simulink model "example"  (R2020a)
settings: Solver=VariableStepAuto  StartTime=0.0  StopTime=stoptime  RelTol=1e-3
values from neighbouring files (symbols this model uses):
  Input_th = [pi/4 0]    [data.m]
libraries: dspfdesign x5
settings Model: Creator=SURAJ  LastModifiedBy=shita
settings DataIOCC: ReturnWorkspaceOutputs=off
settings DebuggingCC: ArithmeticOperatorsInVariantConditions=warning
settings SFSimCC: SimUseLocalCustomCode=off  CustomCodeUndefinedFunction=UseInterfaceOnly
settings RTWCC: RTWUseLocalCustomCode=off

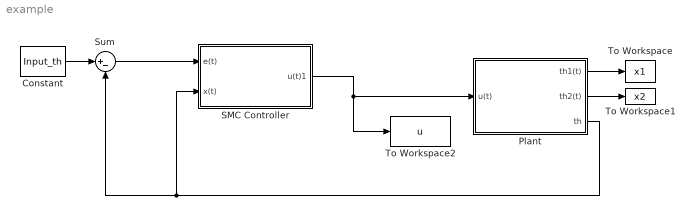
== system example ==
  Constant : Constant  Value=Input_th
  Plant : Subsystem
  SMC Controller : Subsystem
  Sum : Sum  Inputs=|+-
  To Workspace : ToWorkspace  VariableName=x1  SaveFormat=Timeseries  SampleTime=-1
  To Workspace1 : ToWorkspace  VariableName=x2  SaveFormat=Timeseries  SampleTime=-1
  To Workspace2 : ToWorkspace  VariableName=u  SaveFormat=Timeseries  SampleTime=-1
  wires:
  Plant/3(th) -> Sum/2, SMC Controller/2(x(t))
  Plant/1(th1(t)) -> To Workspace/1
  Plant/2(th2(t)) -> To Workspace1/1
  SMC Controller/1(u(t)1) -> To Workspace2/1, Plant/1(u(t))
  Constant/1 -> Sum/1
  Sum/1 -> SMC Controller/1(e(t))

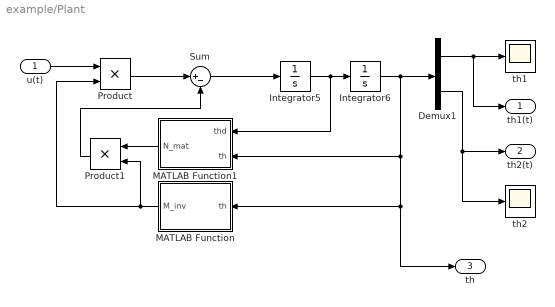
== system example/Plant ==
  u(t) : Inport
  Demux1 : Demux  Outputs=2
  Integrator5 : Integrator
  Integrator6 : Integrator
  MATLAB Function : MATLAB Function  TreatAsAtomicUnit=on
  MATLAB Function1 : MATLAB Function  TreatAsAtomicUnit=on
  Product : Product
  Product1 : Product
  Sum : Sum  Inputs=|+-
  th1 : Scope
  th2 : Scope
  th1(t) : Outport  VectorParamsAs1DForOutWhenUnconnected=off
  th2(t) : Outport  Port=2  VectorParamsAs1DForOutWhenUnconnected=off
  th : Outport  Port=3  VectorParamsAs1DForOutWhenUnconnected=off
  wires:
  u(t)/1 -> Product/1
  Sum/1 -> Integrator5/1
  Demux1/1 -> th1(t)/1, th1/1
  Product1/1 -> Sum/2
  MATLAB Function1/1(N_mat) -> Product1/1
  MATLAB Function/1(M_inv) -> Product1/2, Product/2
  Integrator6/1 -> th/1, MATLAB Function/1(th), MATLAB Function1/2(th), Demux1/1
  Product/1 -> Sum/1
  Demux1/2 -> th2(t)/1, th2/1
  Integrator5/1 -> Integrator6/1, MATLAB Function1/1(thd)

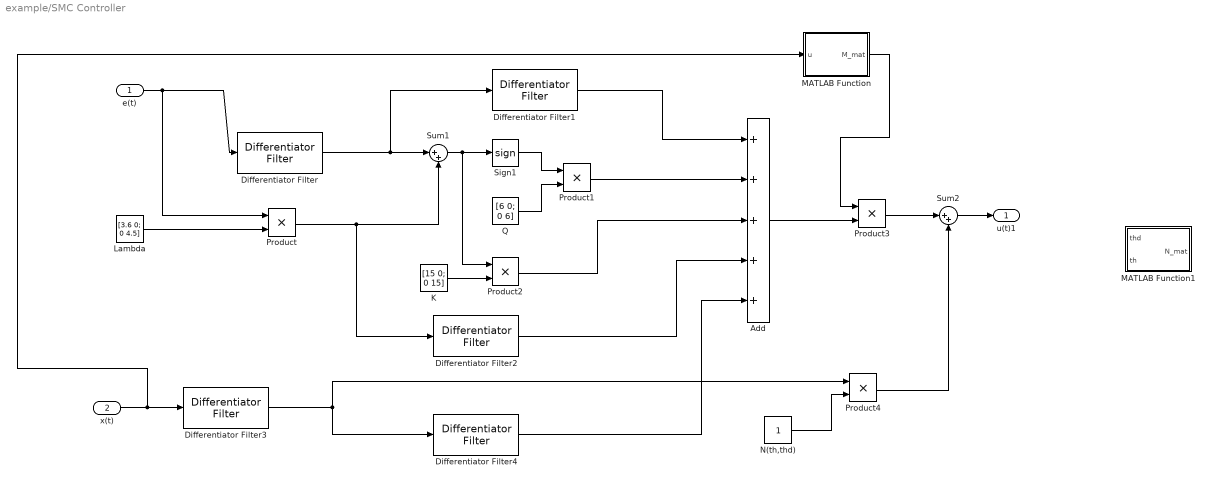
== system example/SMC Controller ==
  e(t) : Inport
  x(t) : Inport  Port=2
  Add : Sum  Inputs=+++++
  Differentiator Filter{,1..4} (5 alike) : dspfdesign/Differentiator Filter  DesignForMinimumOrder=on  FilterOrder=31  PassbandRipple=0.1  ScaleCoefficients=off  SimulateUsing=Interpreted execution  roundingMode=Floor  coeffsDataTypeStr=fixdt(1,16)
      settings: SourceProductBaseCode=DS
  K : Constant  Value=[15 0; 0 15]  VectorParams1D=off
  Lambda : Constant  Value=[3.6 0; 0 4.5]  VectorParams1D=off
  MATLAB Function : MATLAB Function  TreatAsAtomicUnit=on
  MATLAB Function1 : MATLAB Function  TreatAsAtomicUnit=on
  N(th,thd) : Constant
  Product{,1..4} (5 alike) : Product
  Q : Constant  Value=[6 0; 0 6]  VectorParams1D=off
  Sign1 : Signum  ZeroCross=off
  Sum1 : Sum  Inputs=|++
  Sum2 : Sum  Inputs=|++
  u(t)1 : Outport  VectorParamsAs1DForOutWhenUnconnected=off
  wires:
  Differentiator Filter/1 -> Differentiator Filter1/1, Sum1/1
  e(t)/1 -> Differentiator Filter/1, Product/1
  Lambda/1 -> Product/2
  Differentiator Filter1/1 -> Add/1
  Sum1/1 -> Product2/1, Sign1/1
  Sign1/1 -> Product1/1
  Product1/1 -> Add/2
  Q/1 -> Product1/2
  Product/1 -> Differentiator Filter2/1, Sum1/2
  K/1 -> Product2/2
  Product2/1 -> Add/3
  Differentiator Filter2/1 -> Add/4
  Add/1 -> Product3/2
  MATLAB Function/1(M_mat) -> Product3/1
  x(t)/1 -> Differentiator Filter3/1, MATLAB Function/1(u)
  Differentiator Filter3/1 -> Product4/1, Differentiator Filter4/1
  N(th,thd)/1 -> Product4/2
  Product4/1 -> Sum2/2
  Differentiator Filter4/1 -> Add/5
  Product3/1 -> Sum2/1
  Sum2/1 -> u(t)1/1

== matlab function example/SMC Controller/MATLAB Function ==
  data: u input; M_mat output
function M_mat = Mass_mat(u)
m1 = 20;
m2 = 10;
L1 = 0.5;
L2 = 0.5;
a1 = 0.5;
a2 = 0.5;
I1 = 0.8;
I2 = 0.2;
th2 = u(2);
M11 = I1 + m1*L1*L1 + I2 + m2*(a1*a1 + L2*L2 + 2*a1 * L2 * cos(th2));
M12 = I2 + m2 * (L2 * L2 + a1 * L2 * cos(th2));
M21 = M12;
M22 = I2 + m2*L2*L2;
M_mat = [M11 M12; M21 M22];

== matlab function example/Plant/MATLAB Function ==
  data: th input; M_inv output
function M_inv = Mass_mat(th)
th2 = th(2);
m1 = 20;
m2 = 10;
L1 = 0.5;
L2 = 0.5;
a1 = 0.5;
a2 = 0.5;
I1 = 0.8;
I2 = 0.2;
M11 = I1 + m1*L1*L1 + I2 + m2*(a1*a1 + L2*L2 + 2*a1 * L2 * cos(th2));
M12 = I2 + m2 * (L2 * L2 + a1 * L2 * cos(th2));
M21 = M12;
M22 = I2 + m2*L2*L2;
M_mat = [M11 M12; M21 M22];
M_inv = inv(M_mat);

== matlab function example/Plant/MATLAB Function1 ==
  data: thd input; th input; N_mat output
function N_mat= N_func(thd, th)
th1 = th(1);
th2 = th(2);
th1d = thd(1);
th2d = thd(2);
m1 = 20;
m2 = 10;
L1 = 0.5;
L2 = 0.5;
a1 = 0.5;
a2 = 0.5;
N11 = -m2 * a2 * L2 * th1d * sin(th2);
N12 = -m2* a1 * L2*(th1d + th2d)*sin(th2);
N21 = m2*a1*th1d*sin(th2);
N_mat = [(N11*th1d)+(N12*th2d) N21*(th1d)];

== matlab function example/SMC Controller/MATLAB Function1 ==
  data: thd input; N_mat output; th input
function N_mat= N_func(thd, th)
th1 = th(1);
th2 = th(2);
th1d = thd(1);
th2d = thd(2);
m1 = 20;
m2 = 10;
L1 = 0.5;
L2 = 0.5;
a1 = 0.5;
a2 = 0.5;
N11 = -m2 * a2 * L2 * th1d * sin(th2);
N12 = -m2* a1 * L2*(th1d + th2d)*sin(th2);
N21 = m2*a1*th1d*sin(th2);
N_mat = [(N11*th1d)+(N12*th2d) N21*(th1d)];
